simulink model "Registro_Harness_Test1"  (R2020a)
settings: Solver=VariableStepAuto  StartTime=0.0  StopTime=10.0  RelTol=1e-3
settings Model: DataDictionary=Registro_variables.sldd  Creator=Juan  LastModifiedBy=Juan

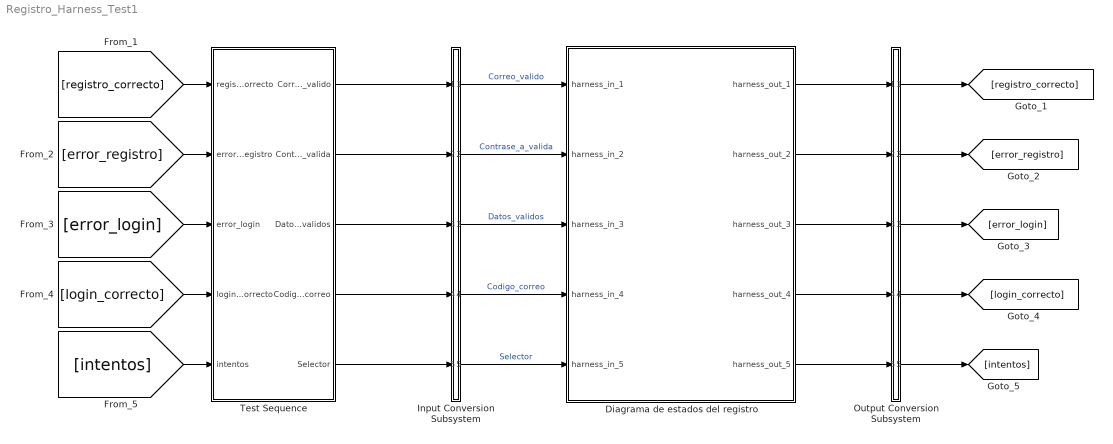
== system Registro_Harness_Test1 ==
  Diagrama de estados del registro : Subsystem  Tag=__SL_testing_harness_stub_
  Input Conversion Subsystem : Subsystem  Tag=__SLT_ICS__  Description=|
      | Signal spec.
      | and routing
      settings: AttributesFormatString=%<Description>
  Output Conversion Subsystem : Subsystem  Tag=__SLT_OCS__  Description=|
      | Signal spec.
      | and routing
      settings: AttributesFormatString=%<Description>
  Test Sequence : Test Sequence  TreatAsAtomicUnit=on
  wires:
  Test Sequence/1(Correo_valido) -> Input Conversion Subsystem/1(Inport_1)
  Test Sequence/2(Contrase_a_valida) -> Input Conversion Subsystem/2(Inport_2)
  Test Sequence/3(Datos_validos) -> Input Conversion Subsystem/3(Inport_3)
  Test Sequence/4(Codigo_correo) -> Input Conversion Subsystem/4(Inport_4)
  Test Sequence/5(Selector) -> Input Conversion Subsystem/5(Inport_5)
  [registro_correcto] -> Test Sequence/1(registro_correcto)
  [error_registro] -> Test Sequence/2(error_registro)
  [error_login] -> Test Sequence/3(error_login)
  [login_correcto] -> Test Sequence/4(login_correcto)
  [intentos] -> Test Sequence/5(intentos)
  Output Conversion Subsystem/1(Outport_1) -> [registro_correcto]
  Output Conversion Subsystem/2(Outport_2) -> [error_registro]
  Output Conversion Subsystem/3(Outport_3) -> [error_login]
  Output Conversion Subsystem/4(Outport_4) -> [login_correcto]
  Output Conversion Subsystem/5(Outport_5) -> [intentos]
  Input Conversion Subsystem/1(Outport_1) -> Diagrama de estados del registro/1(harness_in_1)  "Correo_valido"
  Input Conversion Subsystem/2(Outport_2) -> Diagrama de estados del registro/2(harness_in_2)  "Contrase_a_valida"
  Input Conversion Subsystem/3(Outport_3) -> Diagrama de estados del registro/3(harness_in_3)  "Datos_validos"
  Input Conversion Subsystem/4(Outport_4) -> Diagrama de estados del registro/4(harness_in_4)  "Codigo_correo"
  Input Conversion Subsystem/5(Outport_5) -> Diagrama de estados del registro/5(harness_in_5)  "Selector"
  Diagrama de estados del registro/1(harness_out_1) -> Output Conversion Subsystem/1(Inport_1)
  Diagrama de estados del registro/2(harness_out_2) -> Output Conversion Subsystem/2(Inport_2)
  Diagrama de estados del registro/3(harness_out_3) -> Output Conversion Subsystem/3(Inport_3)
  Diagrama de estados del registro/4(harness_out_4) -> Output Conversion Subsystem/4(Inport_4)
  Diagrama de estados del registro/5(harness_out_5) -> Output Conversion Subsystem/5(Inport_5)

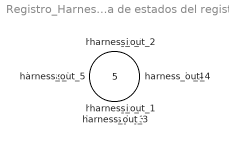
== system Registro_Harness_Test1/Diagrama de estados del registro ==
  harness_in_1 : Inport
  harness_in_2 : Inport  Port=2
  harness_in_3 : Inport  Port=3
  harness_in_4 : Inport  Port=4
  harness_in_5 : Inport  Port=5
  harness_out_1 : Outport
  harness_out_2 : Outport  Port=2
  harness_out_3 : Outport  Port=3
  harness_out_4 : Outport  Port=4
  harness_out_5 : Outport  Port=5

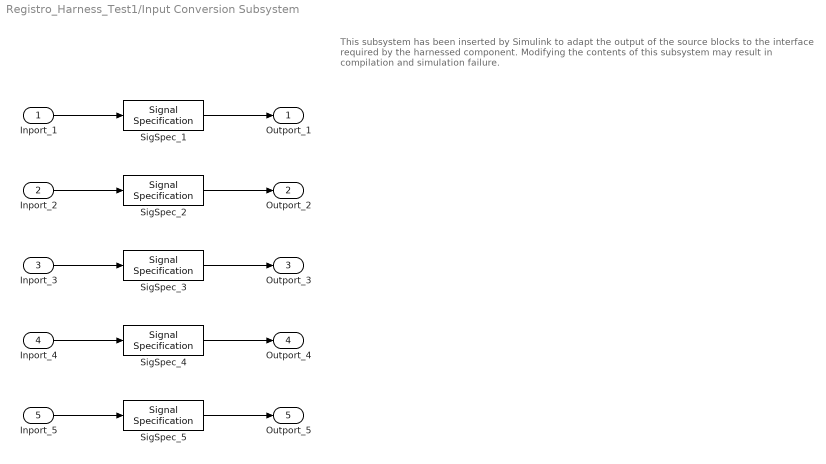
== system Registro_Harness_Test1/Input Conversion Subsystem ==
  note: This subsystem has been inserted by Simulink to adapt the output of the source blocks to the interface required by the harnessed component.
      |  Modifying the contents of this subsystem may result in compilation and simulation failure.
  Inport_1 : Inport
  Inport_2 : Inport  Port=2
  Inport_3 : Inport  Port=3
  Inport_4 : Inport  Port=4
  Inport_5 : Inport  Port=5
  SigSpec_{1..4} (4 alike) : SignalSpecification  OutDataTypeStr=boolean  Dimensions=[1]  SampleTime=[-1, 0]
  SigSpec_5 : SignalSpecification  OutDataTypeStr=fixdt('int64')  Dimensions=[1]  SampleTime=[-1, 0]
  Outport_1 : Outport
  Outport_2 : Outport  Port=2
  Outport_3 : Outport  Port=3
  Outport_4 : Outport  Port=4
  Outport_5 : Outport  Port=5
  wires:
  SigSpec_1/1 -> Outport_1/1
  Inport_1/1 -> SigSpec_1/1
  SigSpec_2/1 -> Outport_2/1
  Inport_2/1 -> SigSpec_2/1
  SigSpec_3/1 -> Outport_3/1
  Inport_3/1 -> SigSpec_3/1
  SigSpec_4/1 -> Outport_4/1
  Inport_4/1 -> SigSpec_4/1
  SigSpec_5/1 -> Outport_5/1
  Inport_5/1 -> SigSpec_5/1

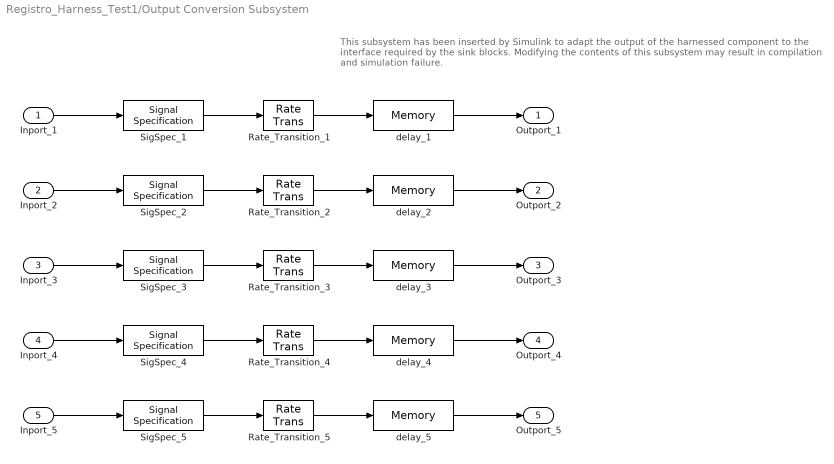
== system Registro_Harness_Test1/Output Conversion Subsystem ==
  note: This subsystem has been inserted by Simulink to adapt the output of the harnessed component to the interface required by the sink blocks.
      |  Modifying the contents of this subsystem may result in compilation and simulation failure.
  Inport_1 : Inport
  Inport_2 : Inport  Port=2
  Inport_3 : Inport  Port=3
  Inport_4 : Inport  Port=4
  Inport_5 : Inport  Port=5
  Rate_Transition_{1..5} (5 alike) : RateTransition  OutPortSampleTimeOpt=Inherit
  SigSpec_{1..4} (4 alike) : SignalSpecification  OutDataTypeStr=boolean  Dimensions=[1]
  SigSpec_5 : SignalSpecification  OutDataTypeStr=fixdt('int64')  Dimensions=[1]
  delay_{1..5} (5 alike) : Memory
  Outport_1 : Outport
  Outport_2 : Outport  Port=2
  Outport_3 : Outport  Port=3
  Outport_4 : Outport  Port=4
  Outport_5 : Outport  Port=5
  wires:
  Inport_1/1 -> SigSpec_1/1
  SigSpec_1/1 -> Rate_Transition_1/1
  Rate_Transition_1/1 -> delay_1/1
  delay_1/1 -> Outport_1/1
  Inport_2/1 -> SigSpec_2/1
  SigSpec_2/1 -> Rate_Transition_2/1
  Rate_Transition_2/1 -> delay_2/1
  delay_2/1 -> Outport_2/1
  Inport_3/1 -> SigSpec_3/1
  SigSpec_3/1 -> Rate_Transition_3/1
  Rate_Transition_3/1 -> delay_3/1
  delay_3/1 -> Outport_3/1
  Inport_4/1 -> SigSpec_4/1
  SigSpec_4/1 -> Rate_Transition_4/1
  Rate_Transition_4/1 -> delay_4/1
  delay_4/1 -> Outport_4/1
  Inport_5/1 -> SigSpec_5/1
  SigSpec_5/1 -> Rate_Transition_5/1
  Rate_Transition_5/1 -> delay_5/1
  delay_5/1 -> Outport_5/1

== stateflow chart Registro_Harness_Test1/Test Sequence ==
  settings: updateMethod=DISCRETE  sampleTime=0.2  stateMachineType=SIMPLIFIED_MACHINE
  state Run
    %% Initialize data outputs.s
    Selector = 1; % fixed-point
  state registro_paso1
    Correo_valido = false;
  state registro_paso2
    Contrase_a_valida = true;
  state registro_paso3
    Datos_validos = true;
  state registro_paso4
    Codigo_correo = true;
  (default) -> Run
  Run -> registro_paso1 : [
      | after(5,sec)
      | ]
  registro_paso1 -> (junction 44) : [
      | after(5,sec)
      | ]
  (junction 44) -> (junction 42)
  registro_paso2 -> registro_paso3 : [
      | after(5,sec)
      | ]
  (junction 42) -> registro_paso3
  registro_paso3 -> registro_paso4 : [
      | after(5,sec)
      | ]
  registro_paso4 -> registro_paso3 : [
      | after(15,sec)
      | ]
  data: registro_correcto input boolean size=[1]; error_registro input boolean size=[1]; error_login input boolean size=[1]; login_correcto input boolean size=[1]; intentos input fixdt('int64') size=[1]; Correo_valido output boolean size=[1]; Contrase_a_valida output boolean size=[1]; Datos_validos output boolean size=[1]; Codigo_correo output boolean size=[1]; Selector output fixdt('int64') size=[1]
